simulink model "antiWindup3"  (R2021a)
settings: Solver=VariableStepAuto  StartTime=0.0  StopTime=10.0  RelTol=1e-3
model workspace (MAT data in the model file):
  Kd = 0.0417
  Ki = 1.06
  Kp = 1
  Threshold = 0.5
undefined symbols (not defined in the file or in its folder): DiscIntNeverNeededParam
libraries: simulink x2
settings Model: Creator=治愈系的小木公子  LastModifiedBy=治愈系的小木公子

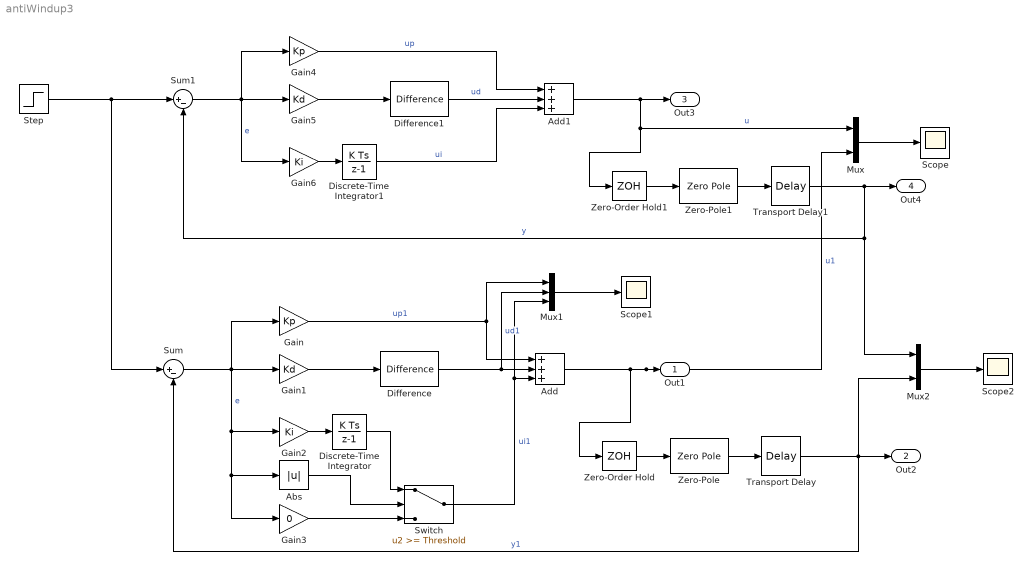
== system antiWindup3 ==
  Abs : Abs
  Add : Sum  Inputs=+++
  Add1 : Sum  Inputs=+++
  Difference : simulink/Discrete/Difference  ICPrevInput=0.0  OutMin=[]  OutMax=[]  OutDataType=fixdt(1, 16)  OutScaling=2^-10  DoSatur=off
  Difference1 : simulink/Discrete/Difference  ICPrevInput=0.0  OutMin=[]  OutMax=[]  OutDataType=fixdt(1, 16)  OutScaling=2^-10  DoSatur=off
  Discrete-Time Integrator : DiscreteIntegrator  SampleTime=0.01  ICPrevOutput=DiscIntNeverNeededParam  ICPrevScaledInput=DiscIntNeverNeededParam
  Discrete-Time Integrator1 : DiscreteIntegrator  SampleTime=0.01  ICPrevOutput=DiscIntNeverNeededParam  ICPrevScaledInput=DiscIntNeverNeededParam
  Gain : Gain  Gain=Kp
  Gain1 : Gain  Gain=Kd
  Gain2 : Gain  Gain=Ki
  Gain3 : Gain  Gain=0
  Gain4 : Gain  Gain=Kp
  Gain5 : Gain  Gain=Kd
  Gain6 : Gain  Gain=Ki
  Mux : Mux  Inputs=2
  Mux1 : Mux  Inputs=3
  Mux2 : Mux  Inputs=2
  Scope : Scope
  Scope1 : Scope
  Scope2 : Scope
  Step : Step  SampleTime=0
  Sum : Sum  Inputs=|+-
  Sum1 : Sum  Inputs=|+-
  Switch : Switch  Threshold=Threshold
  Transport Delay : TransportDelay  DelayTime=0.1
  Transport Delay1 : TransportDelay  DelayTime=0.1
  Zero-Order Hold : ZeroOrderHold  SampleTime=0.01
  Zero-Order Hold1 : ZeroOrderHold  SampleTime=0.01
  Zero-Pole : ZeroPole  Zeros=[]  Poles=[0 -10]  Gain=10
  Zero-Pole1 : ZeroPole  Zeros=[]  Poles=[0 -10]  Gain=10
  Out1 : Outport
  Out2 : Outport  Port=2
  Out3 : Outport  Port=3
  Out4 : Outport  Port=4
  wires:
  Sum/1 -> Gain3/1, Abs/1, Gain2/1, Gain/1, Gain1/1  "e"
  Gain2/1 -> Discrete-Time Integrator/1
  Abs/1 -> Switch/2
  Gain1/1 -> Difference/1
  Transport Delay/1 -> Sum/2, Mux2/2, Out2/1  "y1"
  Add/1 -> Mux/2, Out1/1, Zero-Order Hold/1  "u1"
  Zero-Pole/1 -> Transport Delay/1
  Zero-Order Hold/1 -> Zero-Pole/1
  Gain/1 -> Mux1/1, Add/1  "up1"
  Switch/1 -> Mux1/3, Add/3  "ui1"
  Difference/1 -> Add/2, Mux1/2  "ud1"
  Mux/1 -> Scope/1
  Mux1/1 -> Scope1/1
  Gain3/1 -> Switch/3
  Discrete-Time Integrator/1 -> Switch/1
  Step/1 -> Sum/1, Sum1/1
  Mux2/1 -> Scope2/1
  Difference1/1 -> Add1/2  "ud"
  Gain4/1 -> Add1/1  "up"
  Gain6/1 -> Discrete-Time Integrator1/1
  Transport Delay1/1 -> Mux2/1, Sum1/2, Out4/1  "y"
  Add1/1 -> Out3/1, Zero-Order Hold1/1, Mux/1  "u"
  Sum1/1 -> Gain6/1, Gain4/1, Gain5/1  "e"
  Gain5/1 -> Difference1/1
  Zero-Pole1/1 -> Transport Delay1/1
  Zero-Order Hold1/1 -> Zero-Pole1/1
  Discrete-Time Integrator1/1 -> Add1/3  "ui"
